simulink model "Multiuav"  (Simulink 4.00)
settings: Solver=FixedStepDiscrete  StartTime=0.0  StopTime=g_StopTime  FixedStep=g_SampleTime  RelTol=1e-3
undefined symbols (not defined in the file): ATRFunctions, g_AssignmentAlgorithm, g_CommandTurnRadius, g_CoordinationDelayDen, g_DefaultWaypointAltitude, g_EnableTarget, g_EnableVehicle, g_EntityTypes, g_MaxNumberTargets, g_MaxNumberVehicles, g_MaxReassignmentDeltaTime, g_ObjectMessageIDs, g_OptionSaveDataAVDS, g_OptionSaveDataPlot, g_SampleTime, g_SensorRollLimitDeg, g_TargetStates, g_Tasks, g_TypeAssignment, g_VehicleInputFiles, g_VehicleMemory, g_VehicleTypes, g_WaypointDefinitions, g_WaypointTypes
libraries: cooperative x42
(part 1 of 4)
Description:
  | THIS SOFTWARE AND ANY ACCOMPANYING DOCUMENTATION
  | 
  | IS RELEASED "AS IS." THE U.S.GOVERNMENT MAKES NO WARRANTY
  | 
  | OF ANY KIND, EXPRESS OR IMPLIED, CONCERNING THIS SOFTWARE
  | 
  | AND ANY ACCOMPANYING DOCUMENTATION, INCLUDING, WITHOUT
  | 
  | LIMITATION, ANY WARRANTIES OF MERCHANTABILITY OR FITNESS
  | 
  | FOR A PARTICULAR PURPOSE. IN NO EVENT WILL THE U.S.
  | 
  | GOVERNMENT BE LIABLE FOR ANY DAMAGES, INCLUDING ANY LOST
  | 
  | PROFITS, LOST SAVINGS OR OTHER INCIDENTAL OR CONSEQUENTIAL
  | 
  | DAMAGES ARISING OUT OF THE USE, OR INABILITY TO USE,
  | 
  | THIS SOFTWARE OR ANY ACCOMPANYING DOCUMENTATION, EVEN
  | 
  | IF INFORMED IN ADVANCE OF THE POSSIBILITY OF SUCH DAMAGES.
settings Model: Creator=RAS  LastModifiedBy=RasmusSJ  SaveTime=off  SaveOutput=off  ExtModeAutoUpdateStatusClock=off  OptimizeBlockIOStorage=off  BlockReductionOpt=off

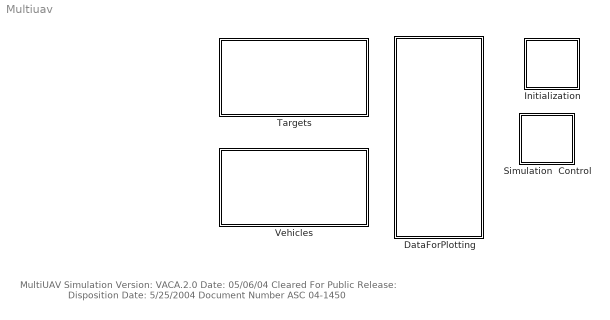
== system Multiuav ==
  note: MultiUAV Simulation
      | Version: VACA.2.0
      | Date: 05/06/04
      | Cleared For Public Release:
      |       Disposition Date: 5/25/2004
      |       Document Number ASC 04-1450
  DataForPlotting : Subsystem  Priority=5
      settings: RTWFcnNameOpts=Auto  RTWFileNameOpts=Auto
  Initialization : Subsystem  Priority=1
      settings: RTWFcnNameOpts=Auto  RTWFileNameOpts=Auto
  Simulation  Control : Subsystem  Priority=10
      settings: RTWFcnNameOpts=Auto  RTWFileNameOpts=Auto
  Targets : Subsystem  Priority=2  TreatAsAtomicUnit=on
      settings: RTWFcnNameOpts=Auto  RTWFileNameOpts=Auto
  Vehicles : Subsystem  Priority=2
      settings: RTWFcnNameOpts=Auto  RTWFileNameOpts=Auto

== system Multiuav/DataForPlotting ==
  note: DataForPlotting
      |
      | PURPOSE: Save vehicle and target state information to text files for
      |      post-simulation plotting.
      |
      | IMPLEMENTATION:
      | - Save Plot Data - when enabled, this subsystem saves the data.
      | - NotAtZero - data saving is enabled when the simulation time is greater
      |      than 0.0 to prevent unitialized data from being written to the file.
      | - EnableDataSaving - reads the global array "OptionSaveDataPlot" to
      |      enable/disable data saving.
  Digital Clock : DigitalClock  SampleTime=g_SampleTime
  Enable Data Saving : Constant  Value=g_OptionSaveDataPlot
  Logical Operator : Logic  Operator=AND  Inputs=2
  NotAtZero : Fcn  Expr=u(1) > 0
  Save Plot Data : Subsystem  TreatAsAtomicUnit=on
      settings: RTWFcnNameOpts=Auto  RTWFileNameOpts=Auto
  wires:
  Logical Operator/1 -> Save Plot Data/Enable
  Enable Data Saving/1 -> Logical Operator/2
  NotAtZero/1 -> Logical Operator/1
  Digital Clock/1 -> NotAtZero/1

== system Multiuav/Initialization ==
  note: Initialization:
      | PURPOSE: This block is used to intialize global variables.
      | IMPLEMENTATION:
      | - Calls the M-Function "InitFunctions.m" to do the initialization.
      | - Only runs during simulation start-up.
      |
      | Simulation Control:
      | PURPOSE: This subsystem is used to invoke functions that
      | allow external control of the simulation.
  note: Simulation Control:
      |
      | PURPOSE: This block is used to invoke functions that
      | allow external control of the simulation.
      | IMPLEMENTATION:
      | - The output of the function block  "ControlTime" set set high when
      | the time is one sample time (g_SampleTime) less than the control
      | time set in the global variable "g_StopTime".
      | - When the ControlTime ouput is high the functions in the
      | block "SimControl" are enabled.
  note: Simulation Control:
      |
      | PURPOSE: This block is used to invoke functions that
      | allow external control of the simulation.
      | IMPLEMENTATION:
      | - When enabled this block calls the function "SimulationControl.m".
  Initialization : S-Function  FunctionName=InitFunctionsS  PortCounts=[]  SFunctionModules=''

== system Multiuav/Simulation  Control ==
  note: Simulation Control:
      |
      | PURPOSE: This block is used to invoke functions that
      | allow external control of the simulation.
      | IMPLEMENTATION:
      | - The output of the function block  "ControlTime" set set high when
      | the time is one sample time (g_SampleTime) less than the control
      | time set in the global variable "g_StopTime".
      | - When the ControlTime ouput is high the functions in the
      | block "SimControl" are enabled.
  SimulationControl : S-Function  FunctionName=SimulationControlS  PortCounts=[]  SFunctionModules=''

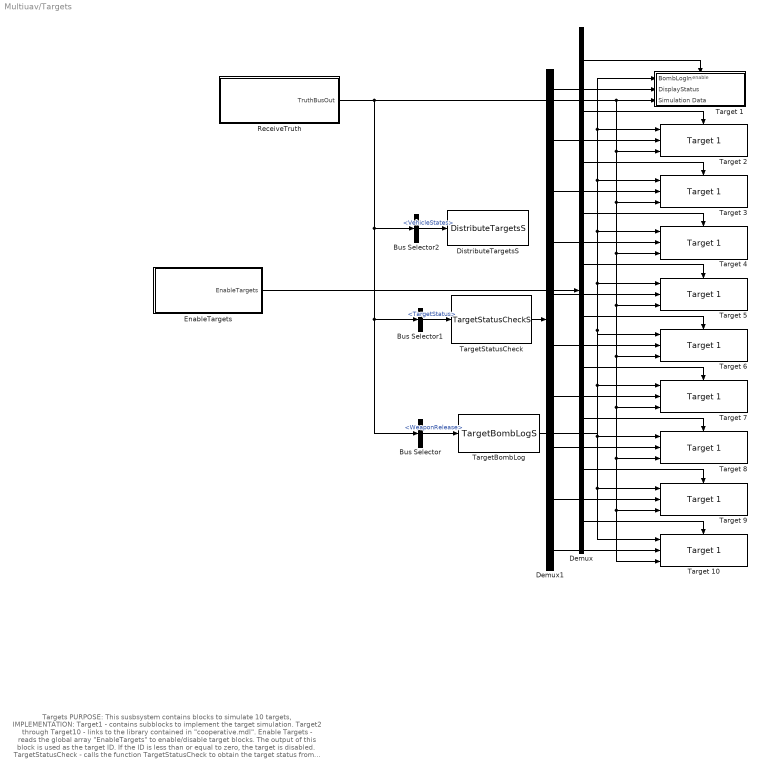
== system Multiuav/Targets ==
  note: Targets
      |
      | PURPOSE: This susbsystem contains blocks to simulate 10 targets,
      |
      | IMPLEMENTATION:
      | Target1 - contains subblocks to implement the target simulation.
      | Target2 through Target10 - links to the library contained in "cooperative.mdl".
      | Enable Targets - reads the global array "EnableTargets" to enable/disable
      |      target blocks. The output of this block is used as the target ID. If the
      |      ID is less than or equal to zero, the target is disabled.
      | TargetStatusCheck - calls the function TargetStatusCheck to obtain the target
      |      status from the vehicles for each of the targets. This is only used to display the
      |      status in plots and AVDS. TargetBombLog - calls the function TargetBombLog
      |      to register any bombs dropped by the vehicles. Each bomb is save with a
      |      unique ID.
      |
      | NOTE: to make changes to the target simulations, first makes changes to
      | the block, "Target1". Next open the library, "cooperative.mdl". Copy the block
      | "Target1" and paste it into "cooperative.mdl". Save "cooperative.mdl".
  Bus Selector : BusSelector  OutputSignals=WeaponRelease  MuxedOutput=on
  Bus Selector1 : BusSelector  OutputSignals=TargetStatus  MuxedOutput=on
  Bus Selector2 : BusSelector  OutputSignals=VehicleStates  MuxedOutput=on
  Demux : Demux  Outputs=g_MaxNumberTargets  BusSelectionMode=off
  Demux1 : Demux  Outputs=g_MaxNumberTargets  BusSelectionMode=off
  DistributeTargetsS : S-Function  FunctionName=DistributeTargetsS  PortCounts=[]  SFunctionModules=''
  EnableTargets : Subsystem
      settings: RTWFcnNameOpts=Auto  RTWFileNameOpts=Auto
  ReceiveTruth : Subsystem
      settings: RTWFcnNameOpts=Auto  RTWFileNameOpts=Auto
  Target 1 : Subsystem  AncestorBlock=cooperative/Target 1  TreatAsAtomicUnit=on
      settings: RTWFcnNameOpts=Auto  RTWFileNameOpts=Auto
  Target {2..10} (9 alike) : cooperative/Target 1  AncestorBlock=cooperative/Target 1  TreatAsAtomicUnit=on
      settings: RTWFcnNameOpts=Auto  RTWFileNameOpts=Auto
  TargetBombLog : S-Function  FunctionName=TargetBombLogS  PortCounts=[]  SFunctionModules=''
  TargetStatusCheck : S-Function  FunctionName=TargetStatusCheckS  PortCounts=[]  SFunctionModules=''
  wires:
  EnableTargets/1(EnableTargets) -> Demux/1
  Demux/1 -> Target 1/Enable
  Demux/2 -> Target 2/Enable
  Demux/3 -> Target 3/Enable
  Demux/4 -> Target 4/Enable
  Demux/5 -> Target 5/Enable
  Demux/6 -> Target 6/Enable
  Demux/7 -> Target 7/Enable
  Demux/8 -> Target 8/Enable
  Demux/9 -> Target 9/Enable
  Demux/10 -> Target 10/Enable
  Bus Selector/1 -> TargetBombLog/1  "<WeaponRelease>"
  TargetBombLog/1 -> Target 9/1, Target 10/1, Target 8/1, Target 7/1, Target 6/1, Target 5/1, Target 4/1, Target 3/1, Target 1/1(BombLogIn), Target 2/1
  Bus Selector1/1 -> TargetStatusCheck/1  "<TargetStatus>"
  TargetStatusCheck/1 -> Demux1/1
  Demux1/1 -> Target 1/2(DisplayStatus)
  Demux1/2 -> Target 2/2
  Demux1/3 -> Target 3/2
  Demux1/4 -> Target 4/2
  Demux1/5 -> Target 5/2
  Demux1/6 -> Target 6/2
  Demux1/7 -> Target 7/2
  Demux1/8 -> Target 8/2
  Demux1/9 -> Target 9/2
  Demux1/10 -> Target 10/2
  Bus Selector2/1 -> DistributeTargetsS/1  "<VehicleStates>"
  ReceiveTruth/1(TruthBusOut) -> Target 1/3(Simulation Data), Target 2/3, Target 3/3, Target 4/3, Target 5/3, Target 6/3, Target 7/3, Target 8/3, Target 9/3, Target 10/3, Bus Selector2/1, Bus Selector/1, Bus Selector1/1

== system Multiuav/Vehicles ==
  note: Vehicles
      |
      | PURPOSE: This susbsystem contains blocks to simulate 8 vehicles,
      |
      | IMPLEMENTATION:
      | UAV1 - contains subblocks to implement the vehicle simulation.
      | UAV2 through UAV8 -links to the library contained in "cooperative.mdl"
      | EnableVehicleID - a subsystem containing logic for enabling vehicle blocks.
      |
      | NOTE: to make changes to the vehicle simulations, first makes changes to
      | the block, "UAV1". Next open the library, "cooperative.mdl". Copy the block
      | "UAV1" and paste it into "cooperative.mdl". Save "cooperative.mdl".
  Demux : Demux  Outputs=g_MaxNumberVehicles  BusSelectionMode=off
  EnableVehiclesID : Subsystem  Priority=1  TreatAsAtomicUnit=on
      settings: RTWFcnNameOpts=Auto  RTWFileNameOpts=Auto
  UAV1 : Subsystem  Priority=2
      settings: RTWFcnNameOpts=Auto  RTWFileNameOpts=Auto
  UAV{2..8} (7 alike) : cooperative/UAV1
      settings: RTWFcnNameOpts=Auto  RTWFileNameOpts=Auto
  wires:
  EnableVehiclesID/1(EnableVehicleID) -> Demux/1
  Demux/1 -> UAV1/1(VehicleID)
  Demux/2 -> UAV2/1
  Demux/3 -> UAV3/1
  Demux/4 -> UAV4/1
  Demux/5 -> UAV5/1
  Demux/6 -> UAV6/1
  Demux/7 -> UAV7/1
  Demux/8 -> UAV8/1

== system Multiuav/DataForPlotting/Save Plot Data ==
  note: SavePlot Data
      |
      | PURPOSE: Saves vehicle and target state information to a text files for use
      |      in post simulation plotting.
  Enable : EnablePort
  Bus Selector : BusSelector  OutputSignals=TargetState  MuxedOutput=off
  Bus Selector1 : BusSelector  OutputSignals=VehicleStateSaveData  MuxedOutput=on
  Bus Selector2 : BusSelector  OutputSignals=TargetStatus  MuxedOutput=on
  Mux2 : Mux  Inputs=2
  RecieveTruth : cooperative/RecieveTruth
      settings: RTWFcnNameOpts=Auto  RTWFileNameOpts=Auto
  RecieverID : Constant  Value=g_ObjectMessageIDs.DataSaveID
  Save Target Data : ToFile  Filename=SimTargetsOut.mat  MatrixName=TargetPositions  SampleTime=g_SampleTime
  Save Vehicle Data : ToFile  Filename=SimPositionsOut.mat  MatrixName=XYPositions  SampleTime=g_SampleTime
  TargetStatusCheckS : S-Function  FunctionName=TargetStatusCheckS  PortCounts=[]  SFunctionModules=''
  wires:
  Mux2/1 -> Save Target Data/1
  Bus Selector/1 -> Mux2/1  "<TargetState>"
  Bus Selector2/1 -> TargetStatusCheckS/1  "<TargetStatus>"
  TargetStatusCheckS/1 -> Mux2/2
  RecieveTruth/1 -> Bus Selector1/1, Bus Selector/1, Bus Selector2/1
  Bus Selector1/1 -> Save Vehicle Data/1  "<VehicleStateSaveData>"
  RecieverID/1 -> RecieveTruth/1

== system Multiuav/Targets/EnableTargets ==
  note: This block generates the signals that enable/disable the targets.
      | The switch is used to enable the targets for one time step in order
      | to set the default positions for the targets not used in the simulation
  Constant : Constant  Value=0
  Digital Clock : DigitalClock  SampleTime=g_SampleTime
  Enable All Targets : Constant  Value=[1:g_MaxNumberTargets]
  Enable Selected Targets : Constant  Value=g_EnableTarget
  Relational Operator1 : RelationalOperator  Operator===
  Switch : Switch  Threshold=0.5
  Unit Delay : UnitDelay  X0=0  SampleTime=g_SampleTime
      settings: RTWStateStorageClass=Auto
  EnableTargets : Outport  Port=1
  wires:
  Relational Operator1/1 -> Switch/2
  Digital Clock/1 -> Unit Delay/1
  Unit Delay/1 -> Relational Operator1/1
  Constant/1 -> Relational Operator1/2
  Enable All Targets/1 -> Switch/1
  Switch/1 -> EnableTargets/1
  Enable Selected Targets/1 -> Switch/3

== system Multiuav/Targets/ReceiveTruth ==
  note: Communications Bus Simulation
      |
      | PURPOSE: Simulate communication subsystem.
      |
      | IMPLEMENTATION:
      | Vehicle-to-vehicle signals are isolated from the CommBus on CommBusSim.  In the case
      | of delayed communications, this is currently implimented with STL deques in the strigger files.
      | Strigger is essentially a trigger taking an arbitrary vector input that can be armed with a scalar
      | delay value...careful with those "enabled" blocks.
      |
      | See m-files:  GetVehicleCommDelay.m and Initializeg_s.m for the OptionEnableCommDelay.
      |
      | NOTE:  YMMV.
  RecieveTruth : cooperative/RecieveTruth
      settings: RTWFcnNameOpts=Auto  RTWFileNameOpts=Auto
  RecieverID : Constant  Value=g_ObjectMessageIDs.TargetIDFirst
  TruthBusOut : Outport  Port=1
  wires:
  RecieverID/1 -> RecieveTruth/1
  RecieveTruth/1 -> TruthBusOut/1

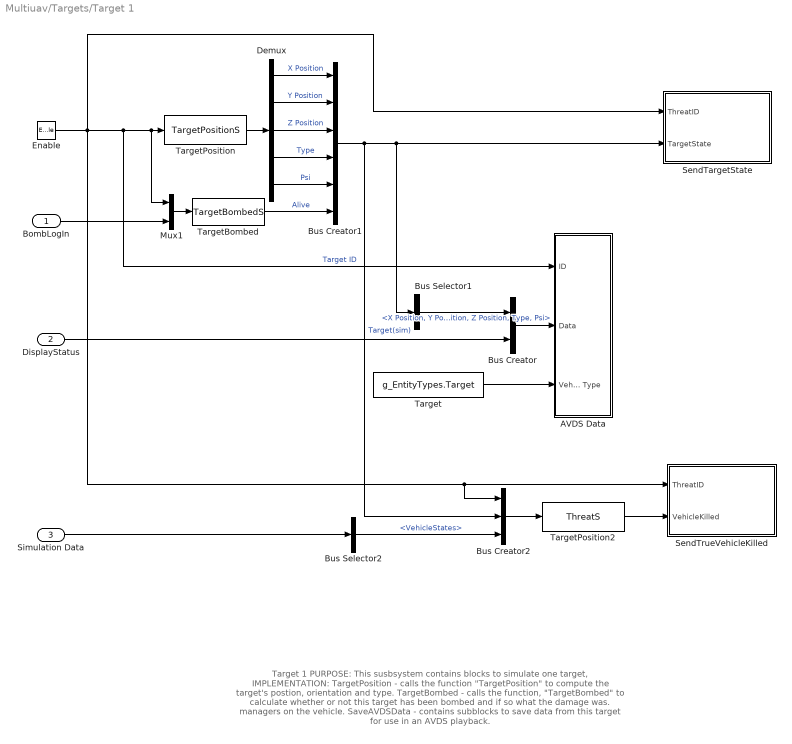
== system Multiuav/Targets/Target 1 ==
  note: Target 1
      |
      | PURPOSE: This susbsystem contains blocks to simulate one target,
      |
      | IMPLEMENTATION:
      | TargetPosition - calls the function "TargetPosition" to compute the target's postion,
      |      orientation and type.
      | TargetBombed - calls the function, "TargetBombed" to calculate whether or not this
      |      target has been bombed and if so what the damage was.
      |      managers on the vehicle.
      | SaveAVDSData - contains subblocks to save data from this target for use
      |     in an AVDS playback.
  BombLogIn : Inport  Port=1  LatchInput=off  SampleTime=g_SampleTime
  DisplayStatus : Inport  Port=2  LatchInput=off  SampleTime=g_SampleTime
  Simulation Data : Inport  Port=3  LatchInput=off  SampleTime=g_SampleTime
  Enable : EnablePort  StatesWhenEnabling=reset  ShowOutputPort=on
  AVDS Data : Subsystem
      settings: RTWFcnNameOpts=Auto  RTWFileNameOpts=Auto
  Bus Creator : BusCreator  Inputs=2
  Bus Creator1 : BusCreator  Inputs=6
  Bus Creator2 : BusCreator  Inputs=3
  Bus Selector1 : BusSelector  OutputSignals=X Position,Y Position,Z Position,Type,Psi  MuxedOutput=on
  Bus Selector2 : BusSelector  OutputSignals=VehicleStates  MuxedOutput=on
  Demux : Demux  Outputs=5  BusSelectionMode=off
  Mux1 : Mux  Inputs=2
  SendTargetState : Subsystem
      settings: RTWFcnNameOpts=Auto  RTWFileNameOpts=Auto
  SendTrueVehicleKilled : Subsystem
      settings: RTWFcnNameOpts=Auto  RTWFileNameOpts=Auto
  Target : Constant  Value=g_EntityTypes.Target
  TargetBombed : S-Function  FunctionName=TargetBombedS  PortCounts=[]  SFunctionModules=''
  TargetPosition : S-Function  FunctionName=TargetPositionS  PortCounts=[]  SFunctionModules=''
  TargetPosition2 : S-Function  FunctionName=ThreatS  Parameters=g_MaxNumberVehicles  PortCounts=[]  SFunctionModules=''
  wires:
  Enable/1 -> AVDS Data/1(ID), Mux1/1, TargetPosition/1, Bus Creator2/1, SendTrueVehicleKilled/1(ThreatID), SendTargetState/1(ThreatID)  "Target ID"
  TargetPosition/1 -> Demux/1
  Target/1 -> AVDS Data/3(Vehicle Type)
  Bus Selector1/1 -> Bus Creator/1  "<X Position, Y Position, Z Position, Type, Psi>"
  Demux/1 -> Bus Creator1/1  "X Position"
  Demux/2 -> Bus Creator1/2  "Y Position"
  Demux/3 -> Bus Creator1/3  "Z Position"
  Bus Creator1/1 -> Bus Selector1/1, SendTargetState/2(TargetState), Bus Creator2/2  "Target(sim)"
  Demux/5 -> Bus Creator1/5  "Psi"
  BombLogIn/1 -> Mux1/2
  Demux/4 -> Bus Creator1/4  "Type"
  TargetBombed/1 -> Bus Creator1/6  "Alive"
  Mux1/1 -> TargetBombed/1
  Bus Creator/1 -> AVDS Data/2(Data)
  DisplayStatus/1 -> Bus Creator/2
  TargetPosition2/1 -> SendTrueVehicleKilled/2(VehicleKilled)
  Bus Creator2/1 -> TargetPosition2/1
  Bus Selector2/1 -> Bus Creator2/3  "<VehicleStates>"
  Simulation Data/1 -> Bus Selector2/1

== system Multiuav/Vehicles/EnableVehiclesID ==
  note: EnableVehiclesID
      |
      | PURPOSE: Output from this block is the vehicle ID if the ID is <= 0 the the
      |      vehicle is disabled.
      |
      | IMPLEMENTATION:
      | FinishDelay01 through FinishDelay08 - These blocks are used to delay the
      |      "Vehicle Finish" signal for three time steps to give other blocks time to finish
      |      terminal functions.
      | Enable Vehicles - reads vehicle IDs from the global array "EnableVehicles". If
      |      the ID is <= 0  the vehicle is disabled.
  Bus Selector : BusSelector  OutputSignals=VehicleIsDead  MuxedOutput=off
  Enable Vehicles : Constant  Value=g_EnableVehicle
  Logical Operator : Logic  Operator=AND  Inputs=2
  Logical Operator1 : Logic  Operator=NOT  Inputs=1
  NotEnabled : Constant  Value=zeros(g_MaxNumberVehicles,1)
  RecieveTruth : cooperative/RecieveTruth
      settings: RTWFcnNameOpts=Auto  RTWFileNameOpts=Auto
  RecieverID : Constant  Value=g_ObjectMessageIDs.VehicleEnableID
  Switch : Switch  Threshold=0.5
  Unit Delay : UnitDelay  X0=0  SampleTime=g_SampleTime
      settings: RTWStateStorageClass=Auto
  Unit Delay1 : UnitDelay  X0=0  SampleTime=g_SampleTime
      settings: RTWStateStorageClass=Auto
  EnableVehicleID : Outport  Port=1
  wires:
  Enable Vehicles/1 -> Logical Operator/1, Switch/1
  Logical Operator1/1 -> Logical Operator/2
  RecieveTruth/1 -> Bus Selector/1
  Logical Operator/1 -> Switch/2
  NotEnabled/1 -> Switch/3
  Switch/1 -> EnableVehicleID/1
  Unit Delay/1 -> Logical Operator1/1
  RecieverID/1 -> RecieveTruth/1
  Bus Selector/1 -> Unit Delay1/1  "<VehicleIsDead>"
  Unit Delay1/1 -> Unit Delay/1

== system Multiuav/Vehicles/UAV1 ==
  note: UAV1
      |
      | PURPOSE: This susbsystem contains blocks to simulate one vehicle,
      |
      | IMPLEMENTATION:
      | Aircraft Dynamics - contains subblocks to implement the vehicle's dynamics
      |      simulation.
      | Embedded Flight Software - contains subblocks to implement the software
      |      managers on the vehicle.
      | SaveAVDSData - contains subblocks to save data from this ehicle for use
      |     in an AVDS playback.
  VehicleID : Inport  Port=1  LatchInput=off  SampleTime=g_SampleTime
  Aircraft Dynamics : Subsystem  TreatAsAtomicUnit=on
      settings: RTWFcnNameOpts=Auto  RTWFileNameOpts=Auto
  Bus Creator : BusCreator  Inputs=1
  Bus Creator1 : BusCreator  Inputs=4
  Bus Creator4 : BusCreator  Inputs=1
  Digital Clock : DigitalClock  SampleTime=g_SampleTime
  EmbeddedFlightSoftware : Subsystem
      settings: RTWFcnNameOpts=Auto  RTWFileNameOpts=Auto
  ReceiveMessages : Subsystem
      settings: RTWFcnNameOpts=Auto  RTWFileNameOpts=Auto
  ReceiveTruth : Subsystem
      settings: RTWFcnNameOpts=Auto  RTWFileNameOpts=Auto
  SaveAVDSData : Subsystem
      settings: RTWFcnNameOpts=Auto  RTWFileNameOpts=Auto
  SendMessages : Subsystem
      settings: RTWFcnNameOpts=Auto  RTWFileNameOpts=Auto
  SendTruth : Subsystem
      settings: RTWFcnNameOpts=Auto  RTWFileNameOpts=Auto
  wires:
  ReceiveMessages/1(CommBusSim Out) -> SendMessages/3(CommBus), EmbeddedFlightSoftware/2(ComBusIn)
  Digital Clock/1 -> Bus Creator1/2  "Time"
  EmbeddedFlightSoftware/2(ComBusOut) -> Bus Creator1/4
  EmbeddedFlightSoftware/1(SimBusOut) -> Bus Creator/1
  VehicleID/1 -> ReceiveMessages/1(VehicleID), SaveAVDSData/1(ID), EmbeddedFlightSoftware/5(Enable), ReceiveTruth/1(Vehicle ID), Bus Creator1/1, SendMessages/1(VehicleID), SendTruth/1(VehicleID), Aircraft Dynamics/Enable  "VehicleID"
  Bus Creator/1 -> SaveAVDSData/3(SimBusLocalln), EmbeddedFlightSoftware/3(SimBusLocalIn), SendTruth/3(SimmBusLocal)  "SimBusLocal"
  Bus Creator1/1 -> SaveAVDSData/2(ComBusLocalln), EmbeddedFlightSoftware/4(ComBusLocalIn), Aircraft Dynamics/2(ComBusLocalIn), SendMessages/2(CommBusLocal), SendTruth/2(CommBusLocal)  "ComBusLocal"
  Aircraft Dynamics/1(ComBusOut) -> Bus Creator1/3
  Bus Creator4/1 -> Aircraft Dynamics/1(SimBusIn), EmbeddedFlightSoftware/1(SimBusIn)
  ReceiveTruth/1(TruthBusOut) -> Bus Creator4/1

== system Multiuav/Targets/Target 1/AVDS Data ==
  note: AVDS Data
      |
      | PURPOSE: Save target state information to a text file that is suitable
      |      for playback in AVDS.
      |
      | IMPLEMENTATION:
      | - Save Target Data for AVDS - calls the function "AVDSData2WorkSpace"
      |      to save the data.
      | - NotAtZero - data saving is enabled when the simulation time is greater
      |      than 0.0 to prevent unitialized data from being written to the file.
      | - EnableDataSaving - reads the global array "OptionSaveDataAVDS" to
      |      enable/disable data saving.
  ID : Inport  Port=1  LatchInput=off  SampleTime=g_SampleTime
  Data : Inport  Port=2  LatchInput=off  SampleTime=g_SampleTime
  Vehicle Type : Inport  Port=3  LatchInput=off  SampleTime=g_SampleTime
  Digital Clock : DigitalClock  SampleTime=g_SampleTime
  EnableDataSaving : Constant  Value=g_OptionSaveDataAVDS
  Logical Operator : Logic  Operator=AND  Inputs=2
  NotAtZero : Fcn  Expr=u(1) > 0
  SaveTarget  Data for AVDS : Subsystem  TreatAsAtomicUnit=on
      settings: RTWFcnNameOpts=Auto  RTWFileNameOpts=Auto
  wires:
  ID/1 -> SaveTarget  Data for AVDS/2(ID)
  Data/1 -> SaveTarget  Data for AVDS/3(Data)
  Digital Clock/1 -> NotAtZero/1, SaveTarget  Data for AVDS/1(Time)
  Vehicle Type/1 -> SaveTarget  Data for AVDS/4(Vehicle Type)
  NotAtZero/1 -> Logical Operator/2
  Logical Operator/1 -> SaveTarget  Data for AVDS/Enable
  EnableDataSaving/1 -> Logical Operator/1

== system Multiuav/Targets/Target 1/SendTargetState ==
  ThreatID : Inport  Port=1  LatchInput=off
  TargetState : Inport  Port=2  LatchInput=off
  Constant : Constant  Value=0
  CreateTargetState : DataStoreMemory  DataStoreName=TargetState  InitialValue=zeros(6,1)
  Enabled Subsystem : Subsystem  TreatAsAtomicUnit=on
      settings: RTWFcnNameOpts=Auto  RTWFileNameOpts=Auto
  Logical Operator : Logic  Orientation=down  Operator=OR  Inputs=2
  Mux2 : Mux  Inputs=3
  ReadTargetState : DataStoreRead  DataStoreName=TargetState  SampleTime=g_SampleTime
  Relational Operator : RelationalOperator  Operator=~=
  Relational Operator1 : RelationalOperator  Orientation=down  Operator===
  "SendTruth " : cooperative/SendTruth   ReuseMatrix=static  MessageTypeStr=TargetState
  Terminator : Terminator
  Unit Delay : UnitDelay  Orientation=left  X0=0  SampleTime=g_SampleTime
      settings: RTWStateStorageClass=Auto
  wires:
  Relational Operator/1 -> Logical Operator/1
  Enabled Subsystem/1(TimeStamp) -> Unit Delay/1, Mux2/2
  ReadTargetState/1 -> Relational Operator/1
  TargetState/1 -> Enabled Subsystem/1(TargetState), Relational Operator/2, Mux2/3
  ThreatID/1 -> Mux2/1
  Mux2/1 -> "SendTruth "/1
  Logical Operator/1 -> Enabled Subsystem/Enable
  Relational Operator1/1 -> Logical Operator/2
  Constant/1 -> Relational Operator1/1
  Unit Delay/1 -> Relational Operator1/2
  "SendTruth "/1 -> Terminator/1

== system Multiuav/Targets/Target 1/SendTrueVehicleKilled ==
  ThreatID : Inport  Port=1  LatchInput=off
  VehicleKilled : Inport  Port=2  LatchInput=off
  CreateVehicleKilled : DataStoreMemory  DataStoreName=VehicleKilled  InitialValue=zeros(g_MaxNumberVehicles,1)
  Enabled Subsystem : Subsystem  TreatAsAtomicUnit=on
      settings: RTWFcnNameOpts=Auto  RTWFileNameOpts=Auto
  Mux2 : Mux  Inputs=4
  ReadVehicleKilled : DataStoreRead  DataStoreName=VehicleKilled  SampleTime=g_SampleTime
  Recipients : Constant  Value=g_ObjectMessageIDs.AllVehiclesTypeShifted + 1
  Relational Operator : RelationalOperator  Operator=~=
  "SendTruth " : cooperative/SendTruth   ReuseMatrix=growing  MessageTypeStr=ChangeVehicleStatus
  Terminator : Terminator
  wires:
  Mux2/1 -> "SendTruth "/1
  ThreatID/1 -> Mux2/1
  VehicleKilled/1 -> Mux2/3, Relational Operator/2, Enabled Subsystem/1(VehicleKilled)
  ReadVehicleKilled/1 -> Relational Operator/1
  Enabled Subsystem/1(TimeStamp) -> Mux2/2
  Relational Operator/1 -> Enabled Subsystem/Enable
  Recipients/1 -> Mux2/4
  "SendTruth "/1 -> Terminator/1

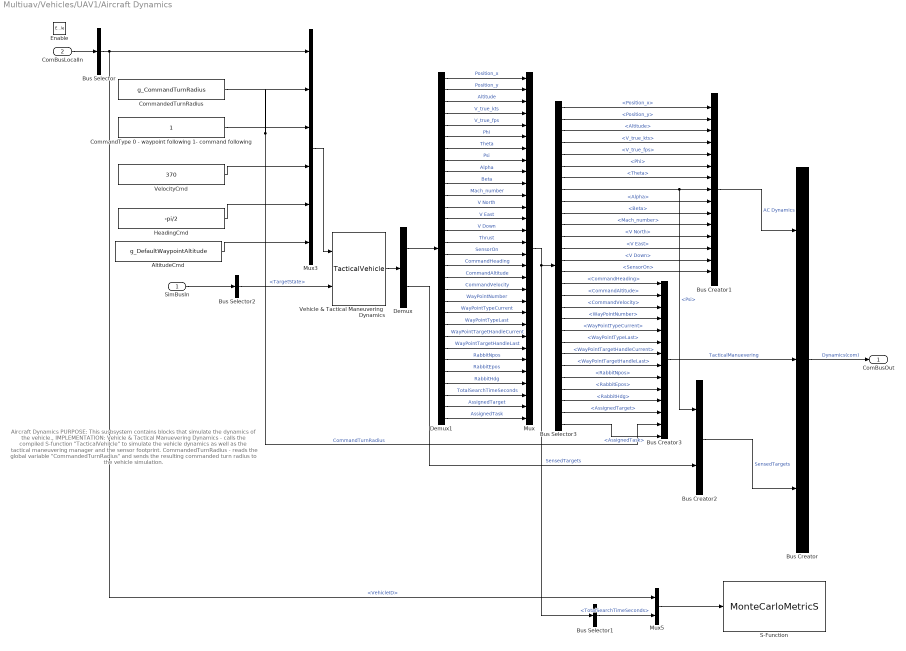
== system Multiuav/Vehicles/UAV1/Aircraft Dynamics ==
  note: Aircraft Dynamics
      |
      | PURPOSE: This susbsystem contains blocks that simulate the dynamics of the vehicle.,
      |
      | IMPLEMENTATION:
      | Vehicle & Tactical Manuevering Dynamics - calls the compiled S-function "TacticalVehilcle"
      |      to simulate the vehicle dynamics as well as the tactical maneuvering manager and the
      |      sensor footprint.
      | CommandedTurnRadius - reads the global variable "CommandedTurnRadius" and sends
      |      the resulting commanded turn radius to the vehicle simulation.
  SimBusIn : Inport  Port=1  LatchInput=off  SampleTime=g_SampleTime
  ComBusLocalIn : Inport  Port=2  LatchInput=off  SampleTime=g_SampleTime
  Enable : EnablePort
  AltitudeCmd : Constant  Value=g_DefaultWaypointAltitude
  Bus Creator : BusCreator  Inputs=3
  Bus Creator1 : BusCreator  Inputs=15
  Bus Creator2 : BusCreator  Inputs=2
  Bus Creator3 : BusCreator  Inputs=14
  Bus Selector : BusSelector  OutputSignals=VehicleID  MuxedOutput=off
  Bus Selector1 : BusSelector  OutputSignals=TotalSearchTimeSeconds  MuxedOutput=off
  Bus Selector2 : BusSelector  OutputSignals=ExternalTruth.TargetState  MuxedOutput=off
  Bus Selector3 : BusSelector  OutputSignals=Position_x,Position_y,Altitude,V_true_kts,V_true_fps,Phi,Theta,Psi,Alpha,Beta,Mach_number,V North,V East,V Down,SensorOn,CommandHeading,CommandAltitude,CommandVelocity,WayPointNumber,WayPointTypeCurrent,WayPointTypeLast,WayPointTargetHandleCurrent,WayPointTargetHandleLast,RabbitNpos,RabbitEpos,RabbitHdg,AssignedTarget,AssignedTask  MuxedOutput=off
  CommandType 0 - waypoint following 1- command following : Constant  Value=1
  CommandedTurnRadius : Constant  Value=g_CommandTurnRadius
  Demux : Demux  Outputs=[30 g_MaxNumberTargets]  BusSelectionMode=off
  Demux1 : Demux  Outputs=30  BusSelectionMode=off
  HeadingCmd : Constant  Value=-pi/2
  Mux : Mux  Inputs=30
  Mux3 : Mux  Inputs=6
  Mux5 : Mux  Inputs=2
  S-Function : S-Function  FunctionName=MonteCarloMetricS  Parameters='TotalSearchTimeSeconds'  PortCounts=[]  SFunctionModules=''
  Vehicle & Tactical Maneuvering  Dynamics : S-Function  FunctionName=TacticalVehicle  Parameters=0,g_MaxNumberTargets,g_SensorRollLimitDeg,g_WaypointDefinitions.NumberEntries,g_VehicleInputFiles  PortCounts=[]  SFunctionModules=''
  VelocityCmd : Constant  Value=370
  ComBusOut : Outport  Port=1
  wires:
  Bus Selector1/1 -> Mux5/2  "<TotalSearchTimeSeconds>"
  Mux5/1 -> S-Function/1
  Demux1/25 -> Mux/25  "RabbitNpos"
  Demux1/30 -> Mux/30  "AssignedTask"
  ComBusLocalIn/1 -> Bus Selector/1
  SimBusIn/1 -> Bus Selector2/1
  Bus Creator3/1 -> Bus Creator/2  "TacticalManuevering"
  Mux/1 -> Bus Selector1/1, Bus Selector3/1
  Bus Selector3/15 -> Bus Creator1/15  "<SensorOn>"
  Bus Creator1/1 -> Bus Creator/1  "AC Dynamics"
  Bus Selector3/14 -> Bus Creator1/14  "<V Down>"
  Bus Selector3/13 -> Bus Creator1/13  "<V East>"
  Bus Selector3/12 -> Bus Creator1/12  "<V North>"
  Bus Selector3/11 -> Bus Creator1/11  "<Mach_number>"
  Bus Selector3/10 -> Bus Creator1/10  "<Beta>"
  Bus Selector3/9 -> Bus Creator1/9  "<Alpha>"
  Bus Selector3/8 -> Bus Creator1/8, Bus Creator2/1  "<Psi>"
  Bus Selector3/7 -> Bus Creator1/7  "<Theta>"
  Bus Selector3/6 -> Bus Creator1/6  "<Phi>"
  Bus Selector3/5 -> Bus Creator1/5  "<V_true_fps>"
  Bus Selector3/4 -> Bus Creator1/4  "<V_true_kts>"
  Bus Selector3/3 -> Bus Creator1/3  "<Altitude>"
  Bus Selector3/2 -> Bus Creator1/2  "<Position_y>"
  Bus Selector3/1 -> Bus Creator1/1  "<Position_x>"
  Demux1/29 -> Mux/29  "AssignedTarget"
  Demux1/27 -> Mux/27  "RabbitHdg"
  Demux1/26 -> Mux/26  "RabbitEpos"
  Demux1/22 -> Mux/22  "WayPointTypeLast"
  Demux1/21 -> Mux/21  "WayPointTypeCurrent"
  Demux1/20 -> Mux/20  "WayPointNumber"
  Demux1/19 -> Mux/19  "CommandVelocity"
  Demux1/18 -> Mux/18  "CommandAltitude"
  Demux1/17 -> Mux/17  "CommandHeading"
  Demux1/16 -> Mux/16  "SensorOn"
  Demux1/15 -> Mux/15  "Thrust"
  Demux1/14 -> Mux/14  "V Down"
  Demux1/13 -> Mux/13  "V East"
  Demux1/12 -> Mux/12  "V North"
  Demux1/11 -> Mux/11  "Mach_number"
  Demux1/10 -> Mux/10  "Beta"
  Demux1/9 -> Mux/9  "Alpha"
  Demux1/8 -> Mux/8  "Psi"
  Demux1/7 -> Mux/7  "Theta"
  Demux1/6 -> Mux/6  "Phi"
  Demux1/5 -> Mux/5  "V_true_fps"
  Demux1/4 -> Mux/4  "V_true_kts"
  Demux1/2 -> Mux/2  "Position_y"
  Demux1/1 -> Mux/1  "Position_x"
  Demux1/3 -> Mux/3  "Altitude"
  Demux/2 -> Bus Creator2/2  "SensedTargets"
  Demux/1 -> Demux1/1
  Bus Creator2/1 -> Bus Creator/3  "SensedTargets"
  Bus Creator/1 -> ComBusOut/1  "Dynamics(com)"
  CommandedTurnRadius/1 -> Bus Creator3/13, Mux3/2  "CommandTurnRadius"
  Bus Selector/1 -> Mux5/1, Mux3/1  "<VehicleID>"
  Vehicle & Tactical Maneuvering  Dynamics/1 -> Demux/1
  Bus Selector2/1 -> Vehicle & Tactical Maneuvering  Dynamics/2  "<TargetState>"
  Mux3/1 -> Vehicle & Tactical Maneuvering  Dynamics/1
  Demux1/23 -> Mux/23  "WayPointTargetHandleCurrent"
  Demux1/24 -> Mux/24  "WayPointTargetHandleLast"
  Demux1/28 -> Mux/28  "TotalSearchTimeSeconds"
  Bus Selector3/16 -> Bus Creator3/1  "<CommandHeading>"
  Bus Selector3/17 -> Bus Creator3/2  "<CommandAltitude>"
  Bus Selector3/18 -> Bus Creator3/3  "<CommandVelocity>"
  Bus Selector3/19 -> Bus Creator3/4  "<WayPointNumber>"
  Bus Selector3/20 -> Bus Creator3/5  "<WayPointTypeCurrent>"
  Bus Selector3/21 -> Bus Creator3/6  "<WayPointTypeLast>"
  Bus Selector3/22 -> Bus Creator3/7  "<WayPointTargetHandleCurrent>"
  Bus Selector3/23 -> Bus Creator3/8  "<WayPointTargetHandleLast>"
  Bus Selector3/24 -> Bus Creator3/9  "<RabbitNpos>"
  Bus Selector3/25 -> Bus Creator3/10  "<RabbitEpos>"
  Bus Selector3/26 -> Bus Creator3/11  "<RabbitHdg>"
  Bus Selector3/27 -> Bus Creator3/12  "<AssignedTarget>"
  Bus Selector3/28 -> Bus Creator3/14  "<AssignedTask>"
  CommandType 0 - waypoint following 1- command following/1 -> Mux3/3
  VelocityCmd/1 -> Mux3/4
  HeadingCmd/1 -> Mux3/5
  AltitudeCmd/1 -> Mux3/6

== system Multiuav/Vehicles/UAV1/EmbeddedFlightSoftware ==
  note: EmbeddedFlightSoftware
      |
      | PURPOSE: This susbsystem contains subsystems to implement the software
      |      managers on the vehicle,
      |
      | IMPLEMENTATION:
      | - Sensor Manager -  This manager is used to perform all of the functions
      |      necessary to monitor the sensors and process sensed data.
      | - TargetManager - Tracks and updates the status of all kown targets.
      | - WeaponsManager - Selects a weapon and then simulates its deployment.
      | - CooperationManager - This manager is used to facilitate cooperation
      |      between the vehicles. At this time the only function implemented is the
      |      Assginment manager.
      | - RouteManager - This manager is used to plan and select the route
      |      for the vehicle to fly. Part of the functionality is calculation of the lowest
      |      cost route to all known targets, based on each target's state.
  SimBusIn : Inport  Port=1  LatchInput=off  SampleTime=g_SampleTime
  ComBusIn : Inport  Port=2  LatchInput=off  SampleTime=g_SampleTime
  SimBusLocalIn : Inport  Port=3  LatchInput=off  SampleTime=g_SampleTime
  ComBusLocalIn : Inport  Port=4  LatchInput=off  SampleTime=g_SampleTime
  Enable : Inport  Port=5  LatchInput=off  SampleTime=g_SampleTime
  Bus Creator : BusCreator  Inputs=3
  Bus Creator1 : BusCreator  Inputs=5
  CooperationManager : Subsystem
      settings: RTWFcnNameOpts=Auto  RTWFileNameOpts=Auto
  RouteManager : Subsystem
      settings: RTWFcnNameOpts=Auto  RTWFileNameOpts=Auto
  SensorManager : Subsystem
      settings: RTWFcnNameOpts=Auto  RTWFileNameOpts=Auto
  TargetManager : Subsystem
      settings: RTWFcnNameOpts=Auto  RTWFileNameOpts=Auto
  TimeLastReplan1 : DataStoreMemory  DataStoreName=TimeLastReplan  InitialValue=0
  WeaponsManager : Subsystem  TreatAsAtomicUnit=on
      settings: RTWFcnNameOpts=Auto  RTWFileNameOpts=Auto
  SimBusOut : Outport  Port=1
  ComBusOut : Outport  Port=2
  wires:
  Enable/1 -> RouteManager/5(Enable), CooperationManager/4(Enable), WeaponsManager/Enable, SensorManager/4(Enable), TargetManager/4(Enable)
  RouteManager/2(ComBusOut) -> Bus Creator1/5
  CooperationManager/1(ComBusOut) -> Bus Creator1/4
  WeaponsManager/2(ComBusOut) -> Bus Creator1/3
  TargetManager/1(ComBusOut) -> Bus Creator1/2
  SensorManager/1(ComBusOut) -> Bus Creator1/1
  RouteManager/1(SimBusOut) -> Bus Creator/3
  WeaponsManager/1(SimBusOut) -> Bus Creator/1
  Bus Creator/1 -> SimBusOut/1  "EFS(sim)"
  Bus Creator1/1 -> ComBusOut/1  "EFS(com)"
  SimBusIn/1 -> TargetManager/1(SimBusIn), SensorManager/1(SimBusIn), CooperationManager/1(SimBusIn), RouteManager/1(SimBusIn)
  ComBusIn/1 -> TargetManager/2(ComBusIn), SensorManager/2(ComBusIn), CooperationManager/2(ComBusIn), RouteManager/2(ComBusIn)
  SimBusLocalIn/1 -> RouteManager/3(SimBusLocalIn)
  ComBusLocalIn/1 -> WeaponsManager/1(ComBusLocalIn), TargetManager/3(ComBusLocalIn), SensorManager/3(ComBusLocalIn), CooperationManager/3(ComBusLocalIn), RouteManager/4(ComBusLocalIn)
  CooperationManager/2(SimBusOut) -> Bus Creator/2

== system Multiuav/Vehicles/UAV1/ReceiveMessages ==
  VehicleID : Inport  Port=1  LatchInput=off
  RecieveCommunications : cooperative/RecieveCommunications
      settings: RTWFcnNameOpts=Auto  RTWFileNameOpts=Auto
  Sum : Sum  Inputs=|++  SaturateOnIntegerOverflow=on
  VehicleOffset : Constant  Value=g_ObjectMessageIDs.VehicleIDOffset
  CommBusSim Out : Outport  Port=1
  wires:
  RecieveCommunications/1 -> CommBusSim Out/1
  VehicleID/1 -> Sum/1
  VehicleOffset/1 -> Sum/2
  Sum/1 -> RecieveCommunications/1

== system Multiuav/Vehicles/UAV1/ReceiveTruth ==
  Vehicle ID : Inport  Port=1  LatchInput=off
  ImplementNewAssignment : Subsystem
      settings: RTWFcnNameOpts=Auto  RTWFileNameOpts=Auto
  RecieveTruth : cooperative/RecieveTruth
      settings: RTWFcnNameOpts=Auto  RTWFileNameOpts=Auto
  Sum : Sum  Inputs=|+|+|  SaturateOnIntegerOverflow=on
  VehicleOffset : Constant  Value=g_ObjectMessageIDs.VehicleIDOffset
  TruthBusOut : Outport  Port=1
  wires:
  RecieveTruth/1 -> TruthBusOut/1, ImplementNewAssignment/2(TruthBus)
  Vehicle ID/1 -> ImplementNewAssignment/1(VehicleID), Sum/2
  Sum/1 -> RecieveTruth/1
  VehicleOffset/1 -> Sum/1

== system Multiuav/Vehicles/UAV1/SaveAVDSData ==
  note: AVDS Data
      |
      | PURPOSE: Save vehicle state information to a
      | text file that is suitable for playback in AVDS.
      |
      | IMPLEMENTATION:
      | - SaveVehicleData for AVDS - calls the function "AVDSData2WorkSpace"
      |      to save the data.
      | - NotAtZero - data saving is enabled when the simulation time is greater
      |      than 0.0 to prevent unitialized data from being written to the file.
      | -EnableDataSaving - reads the global array "OptionSaveDataAVDS" to
      |      enables/disables saving data forAVDS.
  ID : Inport  Port=1  LatchInput=off  SampleTime=g_SampleTime
  ComBusLocalln : Inport  Port=2  LatchInput=off  SampleTime=g_SampleTime
  SimBusLocalln : Inport  Port=3  LatchInput=off  SampleTime=g_SampleTime
  Aircraft : Constant  Value=g_EntityTypes.Aircraft
  Bus Selector2 : BusSelector  OutputSignals=Dynamics(com).AC Dynamics.Position_x,Dynamics(com).AC Dynamics.Position_y,Dynamics(com).AC Dynamics.Altitude,Dynamics(com).AC Dynamics.Phi,Dynamics(com).AC Dynamics.Theta,Dynamics(com).AC Dynamics.Psi,Dynamics(com).AC Dynamics.Alpha,Dynamics(com).AC Dynamics.Beta,Dynamics(com).AC Dynamics.V_true_fps,Dynamics(com).AC Dynamics.Mach_number,Dynamics(com).TacticalManuevering.AssignedTarget,Dynamics(com).TacticalManuevering.AssignedTask,Dynamics(com).TacticalManuevering.RabbitNpos,Dynamics(com).TacticalManuevering.RabbitEpos,Dynamics(com).TacticalManuevering.RabbitHdg,Dynamics(com).TacticalManuevering.CommandAltitude,Dynamics(com).AC Dynamics.SensorOn  MuxedOutput=on
  Bus Selector3 : BusSelector  OutputSignals=EFS(sim).RouteManager(sim).VehicleFinished.Vehicle FinishedNoDelay  MuxedOutput=off
  Digital Clock : DigitalClock  SampleTime=g_SampleTime
  "EnableDataSaving " : Constant  Value=g_OptionSaveDataAVDS
  Logical Operator : Logic  Operator=AND  Inputs=3
  Mux4 : Mux  Inputs=2
  NotAtZero : Fcn  Expr=u(1) > g_SampleTime
  SaveVehicleData for AVDS : Subsystem  TreatAsAtomicUnit=on
      settings: RTWFcnNameOpts=Auto  RTWFileNameOpts=Auto
  wires:
  NotAtZero/1 -> Logical Operator/3
  Aircraft/1 -> SaveVehicleData for AVDS/4(Vehicle Type)
  Digital Clock/1 -> SaveVehicleData for AVDS/1(Time), NotAtZero/1
  SimBusLocalln/1 -> Bus Selector3/1
  ComBusLocalln/1 -> Bus Selector2/1
  ID/1 -> SaveVehicleData for AVDS/2(ID), Logical Operator/2
  Logical Operator/1 -> SaveVehicleData for AVDS/Enable
  "EnableDataSaving "/1 -> Logical Operator/1
  Bus Selector2/1 -> Mux4/1  "<Position_x, Position_y, Altitude, Phi, Theta, Psi, Alpha, Beta, V_true_fps, Mach_number, AssignedTarget, AssignedTask, RabbitNpos, RabbitEpos, RabbitHdg, CommandAltitude, SensorOn>"
  Bus Selector3/1 -> Mux4/2  "<Vehicle FinishedNoDelay>"
  Mux4/1 -> SaveVehicleData for AVDS/3(Data)

== system Multiuav/Vehicles/UAV1/SendMessages ==
  note: Messages must have elements starting with vehicleid,timestamp,...
  VehicleID : Inport  Port=1  LatchInput=off
  CommBusLocal : Inport  Port=2  LatchInput=off
  CommBus : Inport  Port=3  LatchInput=off
  SendATRSingle : Subsystem
      settings: RTWFcnNameOpts=Auto  RTWFileNameOpts=Auto
  SendATRTime : Subsystem
      settings: RTWFcnNameOpts=Auto  RTWFileNameOpts=Auto
  SendAuctionData : Subsystem
      settings: RTWFcnNameOpts=Auto  RTWFileNameOpts=Auto
  SendChangedStatus : Subsystem
      settings: RTWFcnNameOpts=Auto  RTWFileNameOpts=Auto
  SendETAsCostsReturnToSearch : Subsystem
      settings: RTWFcnNameOpts=Auto  RTWFileNameOpts=Auto
  SendPositionFlag : Subsystem
      settings: RTWFcnNameOpts=Auto  RTWFileNameOpts=Auto
  SendPositionID : Subsystem
      settings: RTWFcnNameOpts=Auto  RTWFileNameOpts=Auto
  SendTargetAttacked : Subsystem
      settings: RTWFcnNameOpts=Auto  RTWFileNameOpts=Auto
  SendTargetStatus : Subsystem
      settings: RTWFcnNameOpts=Auto  RTWFileNameOpts=Auto
  SendTaskBenefits : Subsystem
      settings: RTWFcnNameOpts=Auto  RTWFileNameOpts=Auto
  SendTriggerReplan : Subsystem  Priority=1
      settings: RTWFcnNameOpts=Auto  RTWFileNameOpts=Auto
  SendWaypointNumber : Subsystem
      settings: RTWFcnNameOpts=Auto  RTWFileNameOpts=Auto
  wires:
  CommBus/1 -> SendPositionFlag/3(CommBus), SendPositionID/3(CommBus)
  CommBusLocal/1 -> SendATRTime/2(CommBusLocal), SendATRSingle/2(CommBusLocal), SendETAsCostsReturnToSearch/2(CommBusLocal), SendTriggerReplan/2(CommBusLocal), SendAuctionData/2(CommBusLocal), SendTaskBenefits/2(CommBusLocal), SendPositionFlag/2(CommBusLocal), SendPositionID/2(CommBusLocal), SendTargetStatus/2(CommBusLocal), SendTargetAttacked/2(CommBusLocal), SendChangedStatus/2(CommBusLocal), SendWaypointNumber/2(CommBusLocal)
  VehicleID/1 -> SendETAsCostsReturnToSearch/1(VehicleID), SendTriggerReplan/1(VehicleID), SendATRTime/1(VehicleID), SendAuctionData/1(VehicleID), SendTaskBenefits/1(VehicleID), SendPositionFlag/1(VehicleID), SendPositionID/1(VehicleID), SendTargetStatus/1(VehicleID), SendTargetAttacked/1(VehicleID), SendChangedStatus/1(VehicleID), SendWaypointNumber/1(VehicleID), SendATRSingle/1(VehicleID)

== system Multiuav/Vehicles/UAV1/SendTruth ==
  note: Messages must have elements starting with vehicleid,timestamp,...
  VehicleID : Inport  Port=1  LatchInput=off
  CommBusLocal : Inport  Port=2  LatchInput=off
  SimmBusLocal : Inport  Port=3  LatchInput=off
  SendNewAssignment : Subsystem
      settings: RTWFcnNameOpts=Auto  RTWFileNameOpts=Auto
  SendTargetStatus : Subsystem
      settings: RTWFcnNameOpts=Auto  RTWFileNameOpts=Auto
  SendTrackList : Subsystem
      settings: RTWFcnNameOpts=Auto  RTWFileNameOpts=Auto
  SendTrueVehicleState : Subsystem
      settings: RTWFcnNameOpts=Auto  RTWFileNameOpts=Auto
  SendVehicleIsDead : Subsystem
      settings: RTWFcnNameOpts=Auto  RTWFileNameOpts=Auto
  SendWeaponsRelease : Subsystem
      settings: RTWFcnNameOpts=Auto  RTWFileNameOpts=Auto
  VehicleStateSaveData : Subsystem
      settings: RTWFcnNameOpts=Auto  RTWFileNameOpts=Auto
  wires:
  VehicleID/1 -> SendVehicleIsDead/1(VehicleID), SendWeaponsRelease/1(VehicleID), SendTargetStatus/1(VehicleID), VehicleStateSaveData/1(VehicleID), SendTrackList/1(VehicleID), SendTrueVehicleState/1(VehicleID), SendNewAssignment/1(VehicleID)
  CommBusLocal/1 -> SendTrueVehicleState/2(CommBusLocal), SendTargetStatus/2(CommBusLocal), VehicleStateSaveData/2(CommBusLocal), SendTrackList/2(CommBusLocal)
  SimmBusLocal/1 -> SendWeaponsRelease/2(SimmBusLocal), SendVehicleIsDead/2(SimmBusLocal), VehicleStateSaveData/3(SimmBusLocal), SendTrueVehicleState/3(SimmBusLocal), SendNewAssignment/2(SimmBusLocal)

== system Multiuav/Targets/Target 1/AVDS Data/SaveTarget  Data for AVDS ==
  note: SaveTargetData for AVDS
      |
      | PURPOSE: Saves target state information to a text file that is suitable
      |      for playback in AVDS.
      | IMPLEMENTATION:
      | - AVDSData2WorkSpace - calls the M-function "AVDSData2WorkSpace"
      |      to save the data.
  Time : Inport  Port=1  LatchInput=off  SampleTime=g_SampleTime
  ID : Inport  Port=2  LatchInput=off  SampleTime=g_SampleTime
  Data : Inport  Port=3  LatchInput=off  SampleTime=g_SampleTime
  Vehicle Type : Inport  Port=4  LatchInput=off  SampleTime=g_SampleTime
  Enable : EnablePort
  AVDSData2WorkSpaceS : S-Function  FunctionName=AVDSData2WorkSpaceS  PortCounts=[]  SFunctionModules=''
  Mux1 : Mux  Inputs=4
  wires:
  Mux1/1 -> AVDSData2WorkSpaceS/1
  Time/1 -> Mux1/2
  ID/1 -> Mux1/1
  Data/1 -> Mux1/3
  Vehicle Type/1 -> Mux1/4

== system Multiuav/Targets/Target 1/SendTargetState/Enabled Subsystem ==
  TargetState : Inport  Port=1  LatchInput=off
  Enable : EnablePort
  Digital Clock : DigitalClock  SampleTime=g_SampleTime
  SaveTargetState : DataStoreWrite  DataStoreName=TargetState  SampleTime=g_SampleTime
  TimeStamp : Outport  Port=1
  wires:
  Digital Clock/1 -> TimeStamp/1
  TargetState/1 -> SaveTargetState/1

== system Multiuav/Targets/Target 1/SendTrueVehicleKilled/Enabled Subsystem ==
  VehicleKilled : Inport  Port=1  LatchInput=off
  Enable : EnablePort
  Digital Clock : DigitalClock  SampleTime=g_SampleTime
  SaveVehicleKilled : DataStoreWrite  DataStoreName=VehicleKilled  SampleTime=g_SampleTime
  TimeStamp : Outport  Port=1
  wires:
  VehicleKilled/1 -> SaveVehicleKilled/1
  Digital Clock/1 -> TimeStamp/1

== system Multiuav/Vehicles/UAV1/EmbeddedFlightSoftware/CooperationManager ==
  note: Cooperation Manager
      |
      | PURPOSE: This manager is used to facilitate cooperation
      |      between the vehicles. At this time the only function
      |      implemented is the Assginment manager which calculates
      |      vehicle /task assignments.
      |
      | IMPLEMENTATION:
      | - Coordination Timing - adds a time delay before the assignment
      |      calculation to give other vehicles time to generate new plans.
      | - Calculate Assignment - this subsystem contains blocks used to
      |      calculate the vehicle/task assignments. This block is enabled
      |      by the signal "New Plans", after the Coordination Timing delay.
  SimBusIn : Inport  Port=1  LatchInput=off  SampleTime=g_SampleTime
  ComBusIn : Inport  Port=2  LatchInput=off  SampleTime=g_SampleTime
  ComBusLocalIn : Inport  Port=3  LatchInput=off  SampleTime=g_SampleTime
  Enable : Inport  Port=4  LatchInput=off  SampleTime=g_SampleTime
  Bus Creator : BusCreator  Inputs=3
  Bus Creator1 : BusCreator  Inputs=1
  Calculate Assignment : Subsystem  TreatAsAtomicUnit=on
      settings: RTWFcnNameOpts=Auto  RTWFileNameOpts=Auto
  Enable Reassignment : Subsystem
      settings: RTWFcnNameOpts=Auto  RTWFileNameOpts=Auto
  Task List : Subsystem
      settings: RTWFcnNameOpts=Auto  RTWFileNameOpts=Auto
  Terminator : Terminator
  ComBusOut : Outport  Port=1
  SimBusOut : Outport  Port=2
  wires:
  Calculate Assignment/3(AuctionData) -> Bus Creator/3
  Calculate Assignment/2(Algorithm Data) -> Bus Creator/2
  Task List/1(UnassignTaskFlag) -> Terminator/1
  SimBusIn/1 -> Calculate Assignment/3(SimBusIn)
  Enable Reassignment/1(Enable Reassignment) -> Calculate Assignment/Enable
  Enable/1 -> Enable Reassignment/1(Enable)
  ComBusLocalIn/1 -> Task List/1(ComBusLocalIn), Enable Reassignment/2(ComBusLocalIn), Calculate Assignment/1(ComBusLocalIn)  "Local Bus"
  ComBusIn/1 -> Enable Reassignment/3(ComBusIn), Calculate Assignment/2(ComBusIn)
  Calculate Assignment/1(Local Assignment) -> Bus Creator/1  "Assignment"
  Bus Creator/1 -> ComBusOut/1  "CooperationManager(com)"
  Calculate Assignment/4(NewAssignmetTime) -> Bus Creator1/1  "NewAssignmentTime"
  Bus Creator1/1 -> SimBusOut/1  "CooperationManager(com)"

== system Multiuav/Vehicles/UAV1/EmbeddedFlightSoftware/RouteManager ==
  note: Route Manager
      |
      | PURPOSE: This manager is used to plan and select the route for the
      |      vehicle to fly.
      |
      | Implementation:
      | - Replan - when enabled, calculates the lowest cost route to all known targets,
      |      based on each target's state. Replan is enabled If any of the vehicles report
      |      "Task Finished" or if any of the targets change state,
      | - RouteSelection - calls the function "RouteSelection" to implement waypoints
      |      for the route selected for this vehicle during the vehicle/target assignment in
      |      the cooperation manager.
      | - Task Status - monitors the status of the vehicle's assigned task.
  SimBusIn : Inport  Port=1  LatchInput=off  SampleTime=g_SampleTime
  ComBusIn : Inport  Port=2  LatchInput=off  SampleTime=g_SampleTime
  SimBusLocalIn : Inport  Port=3  LatchInput=off  SampleTime=g_SampleTime
  ComBusLocalIn : Inport  Port=4  LatchInput=off  SampleTime=g_SampleTime
  Enable : Inport  Port=5  LatchInput=off  SampleTime=g_SampleTime
  Bus Creator : BusCreator  Inputs=1
  Bus Creator1 : BusCreator  Inputs=3
  Constant : Constant  Value=g_AssignmentAlgorithm
  Constant1 : Constant  Value=g_TypeAssignment.CapTransShip
  Logical Operator : Logic  Operator=AND  Inputs=2
  Relational Operator : RelationalOperator  Operator===
  ReplanSingle : Subsystem
      settings: RTWFcnNameOpts=Auto  RTWFileNameOpts=Auto
  Task Status : Subsystem
      settings: RTWFcnNameOpts=Auto  RTWFileNameOpts=Auto
  SimBusOut : Outport  Port=1
  ComBusOut : Outport  Port=2
  wires:
  Constant1/1 -> Relational Operator/2
  Constant/1 -> Relational Operator/1
  Relational Operator/1 -> Logical Operator/1
  Logical Operator/1 -> ReplanSingle/3(Enable)
  Enable/1 -> Task Status/2(Enable), Logical Operator/2
  ReplanSingle/1(NewPlans) -> Bus Creator1/1
  Bus Creator/1 -> SimBusOut/1  "RouteManager(sim)"
  ComBusIn/1 -> ReplanSingle/1(ComBusIn)
  Task Status/1(Task Status) -> Bus Creator1/3
  Task Status/2(Vehicle Finished) -> Bus Creator/1
  SimBusIn/1 -> ReplanSingle/4(SimBusIn), Task Status/3(SimBusIn)
  ReplanSingle/2(ReplanETAsCosts) -> Bus Creator1/2
  Bus Creator1/1 -> ComBusOut/1  "RouteManager(com)"
  ComBusLocalIn/1 -> Task Status/1(Local (Comm)), ReplanSingle/2(ComBusLocalIn)  "Local Bus"
  SimBusLocalIn/1 -> ReplanSingle/5(SimBusLocalIn)  "Vehicle (Sim)"

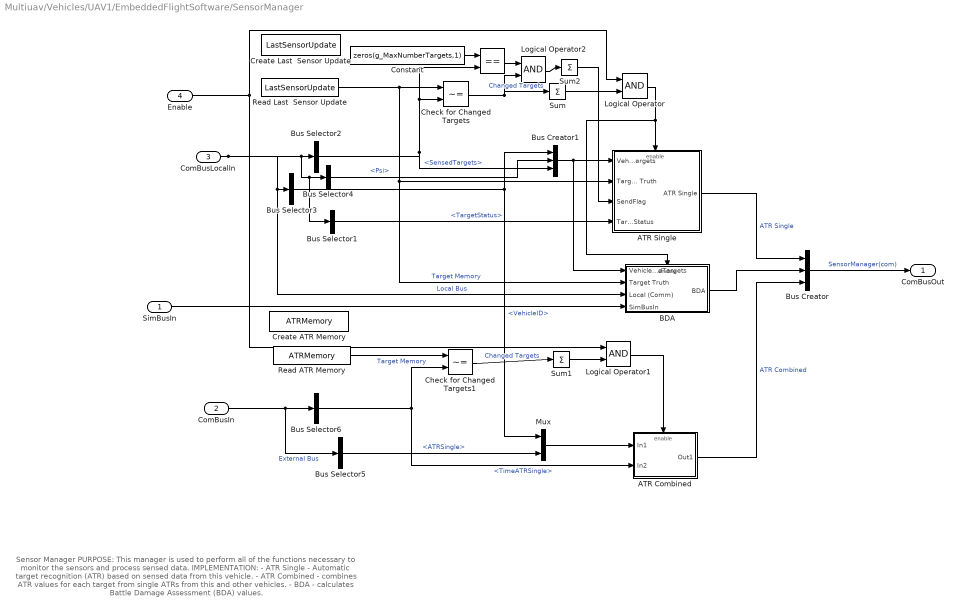
== system Multiuav/Vehicles/UAV1/EmbeddedFlightSoftware/SensorManager ==
  note: Sensor Manager
      |
      | PURPOSE: This manager is used to perform all of the functions
      | necessary to monitor the sensors and process sensed data.
      |
      | IMPLEMENTATION:
      | - ATR Single - Automatic target recognition (ATR) based on sensed data
      |      from this vehicle.
      | - ATR Combined - combines ATR values for each target from single ATRs
      |      from this and other vehicles.
      | - BDA - calculates Battle Damage Assessment (BDA) values.
  SimBusIn : Inport  Port=1  LatchInput=off  SampleTime=g_SampleTime
  ComBusIn : Inport  Port=2  LatchInput=off  SampleTime=g_SampleTime
  ComBusLocalIn : Inport  Port=3  LatchInput=off  SampleTime=g_SampleTime
  Enable : Inport  Port=4  LatchInput=off  SampleTime=g_SampleTime
  " " : RelationalOperator  Operator===
  ATR Combined : Subsystem  TreatAsAtomicUnit=on
      settings: RTWFcnNameOpts=Auto  RTWFileNameOpts=Auto
  ATR Single : Subsystem  TreatAsAtomicUnit=on
      settings: RTWFcnNameOpts=Auto  RTWFileNameOpts=Auto
  BDA : Subsystem  TreatAsAtomicUnit=on
      settings: RTWFcnNameOpts=Auto  RTWFileNameOpts=Auto
  Bus Creator : BusCreator  Inputs=3
  Bus Creator1 : BusCreator  Inputs=3
  Bus Selector1 : BusSelector  OutputSignals=EFS(com).TargetManager(com).Target Status.TargetStatus  MuxedOutput=off
  Bus Selector2 : BusSelector  OutputSignals=Dynamics(com).SensedTargets.SensedTargets  MuxedOutput=off
  Bus Selector3 : BusSelector  OutputSignals=VehicleID  MuxedOutput=off
  Bus Selector4 : BusSelector  OutputSignals=Dynamics(com).AC Dynamics.Psi  MuxedOutput=off
  Bus Selector5 : BusSelector  OutputSignals=ATRSingle  MuxedOutput=off
  Bus Selector6 : BusSelector  OutputSignals=TimeATRSingle  MuxedOutput=off
  Check for Changed Targets : RelationalOperator  Operator=~=
  Check for Changed Targets1 : RelationalOperator  Operator=~=
  Constant : Constant  Value=zeros(g_MaxNumberTargets,1)
  Create ATR Memory : DataStoreMemory  DataStoreName=ATRMemory  InitialValue=1
  Create Last  Sensor Update : DataStoreMemory  DataStoreName=LastSensorUpdate  InitialValue=zeros(g_MaxNumberTargets,1)
  Logical Operator : Logic  Operator=AND  Inputs=2
  Logical Operator1 : Logic  Operator=AND  Inputs=2
  Logical Operator2 : Logic  Operator=AND  Inputs=2
  Mux : Mux  Inputs=2
  Read ATR Memory : DataStoreRead  DataStoreName=ATRMemory  SampleTime=g_SampleTime
  Read Last  Sensor Update : DataStoreRead  DataStoreName=LastSensorUpdate  SampleTime=g_SampleTime
  Sum : Sum  Inputs=|+  SaturateOnIntegerOverflow=on
  Sum1 : Sum  Inputs=|+  SaturateOnIntegerOverflow=on
  Sum2 : Sum  Inputs=|+  SaturateOnIntegerOverflow=on
  ComBusOut : Outport  Port=1
  wires:
  Bus Selector1/1 -> ATR Single/4(TargetStatus)  "<TargetStatus>"
  Sum2/1 -> ATR Single/3(SendFlag)
  Logical Operator2/1 -> Sum2/1
  " "/1 -> Logical Operator2/1
  Constant/1 -> " "/1
  Enable/1 -> Logical Operator1/1, Logical Operator/1
  Logical Operator1/1 -> ATR Combined/Enable
  Sum1/1 -> Logical Operator1/2
  Logical Operator/1 -> BDA/Enable, ATR Single/Enable
  Sum/1 -> Logical Operator/2
  ATR Single/1(ATR Single) -> Bus Creator/1  "ATR Single"
  BDA/1(BDA) -> Bus Creator/2
  Bus Creator/1 -> ComBusOut/1  "SensorManager(com)"
  ATR Combined/1(Out1) -> Bus Creator/3  "ATR Combined"
  Bus Selector6/1 -> ATR Combined/2(In2), Check for Changed Targets1/2  "<TimeATRSingle>"
  Mux/1 -> ATR Combined/1(In1)
  Bus Selector5/1 -> Mux/2  "<ATRSingle>"
  ComBusIn/1 -> Bus Selector5/1, Bus Selector6/1  "External Bus"
  Bus Selector4/1 -> Bus Creator1/2  "<Psi>"
  Bus Selector3/1 -> Mux/1, Bus Creator1/1  "<VehicleID>"
  Bus Selector2/1 -> " "/2, Check for Changed Targets/2, Bus Creator1/3  "<SensedTargets>"
  Bus Creator1/1 -> BDA/1(VehicleID Psi SensedTargets), ATR Single/1(VehicleID Psi SensedTargets)
  ComBusLocalIn/1 -> BDA/3(Local (Comm)), Bus Selector3/1, Bus Selector1/1, Bus Selector4/1, Bus Selector2/1  "Local Bus"
  Read ATR Memory/1 -> Check for Changed Targets1/1  "Target Memory"
  Check for Changed Targets1/1 -> Sum1/1  "Changed Targets"
  Read Last  Sensor Update/1 -> BDA/2(Target Truth), ATR Single/2(Target Truth), Check for Changed Targets/1  "Target Memory"
  Check for Changed Targets/1 -> Logical Operator2/2, Sum/1  "Changed Targets"
  SimBusIn/1 -> BDA/4(SimBusIn)
